simulink model "IEEE_39bus_load_increase_vol1"  (R2024b)
settings: Solver=ode23tb  StartTime=0.0  StopTime=500  MaxStep=1/60  RelTol=1e-2  AbsTol=1e-1  EnableMultiTasking=on
PreLoadFcn:
  | NE39bus_data;
  | PSSMODEL=1;
  | LPSS=0;
  | WAPSS=0;
  | WAPSS2=0;
values from neighbouring files (symbols this model uses):
  deg = [19.62;0;2.466;4.423;3.398;5.698;8.494;2.181;7.784;-3.646]*pi/180    [main_39.m]
  ki_sapc = 0.02*2.5/4    (= 0.0125)    [main_39.m]
  kp = 5*ones(10,1)    [main_39.m]
  kp_sapc = 0.15*1.25    (= 0.1875)    [main_39.m]
  line = [     1	2	0.0035	0.0411	0.6987	0	100	345 ... (first row only)    [main_39.m]
  P_base = mac_con(:,3).*[0.5609;0.6011;0.6995;0.6432;0.5143;0.6634;0.5676;0.5897;0.8444;0.3464]    [main_39.m]
  P_cmd = [1.140 	1.060 	1.100 	1.120 	0	1.060 	1.115 	1.160 	1.175 	1.000 ]    [main_39.m]
  Pmax = [1.20; 1.10; 1.15; 1.15;1.10;1.10;1.15;1.20;1.20;1.00]    [main_39.m]
  Pmin = 2-Pmax    [main_39.m]
  s = 10    [main_39.m]
  ts_pi = 5    [main_39.m]
  Udc = 2*Bus(mac_con(:,2),2)*1e3    [main_39.m]
  V_m = [1.03;0.982;0.9831;0.9972;1.0123;1.0493;1.0635;1.0278;1.0265;1.048]*sqrt(2/3)    [main_39.m]
undefined symbols (not defined in the file or in its folder): D1, Delta
libraries: spsThreePhaseVIMeasurementLib x40, spsThreePhasePISectionLineLib x34, spsThreePhaseParallelRLCLoadLib x21, spsThreePhaseTransformerTwoWindingsLib x13, spsMeanLib x12, slpidlib x12, spsLoadFlowBusLib x10, spsPLL3phLib x10, spsPowerPositiveSequenceLib x10, spsDCVoltageSourceLib x10, simulink x10, spsUniversalBridgeLib x10
(part 2 of 4)

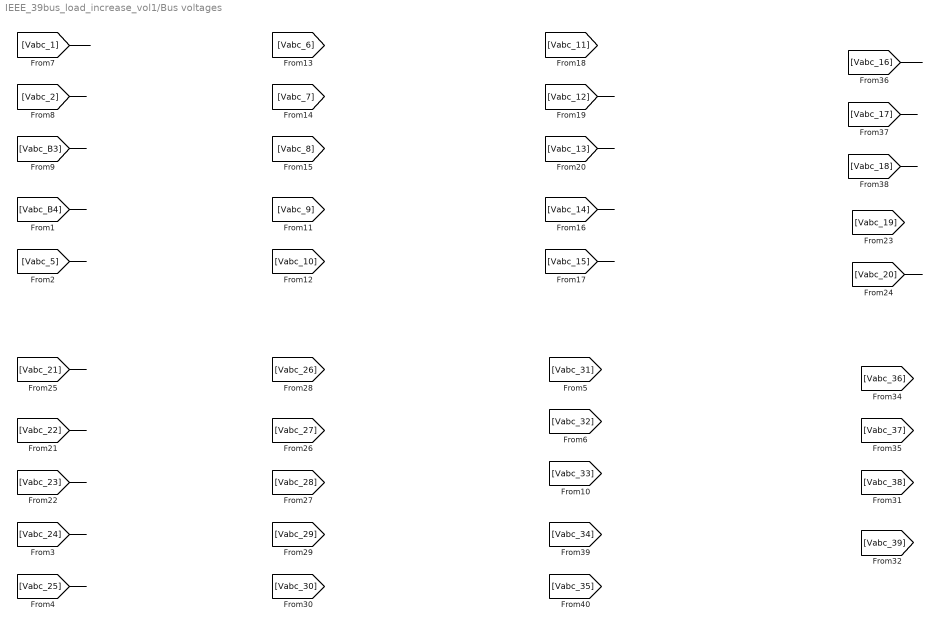
== system IEEE_39bus_load_increase_vol1/Bus voltages ==
  wires:
  [Vabc_1] -> ?
  [Vabc_2] -> ?
  [Vabc_B3] -> ?
  [Vabc_B4] -> ?
  [Vabc_5] -> ?
  [Vabc_24] -> ?
  [Vabc_25] -> ?
  [Vabc_12] -> ?
  [Vabc_13] -> ?
  [Vabc_14] -> ?
  [Vabc_15] -> ?
  [Vabc_20] -> ?
  [Vabc_21] -> ?
  [Vabc_22] -> ?
  [Vabc_23] -> ?
  [Vabc_16] -> ?
  [Vabc_17] -> ?
  [Vabc_18] -> ?

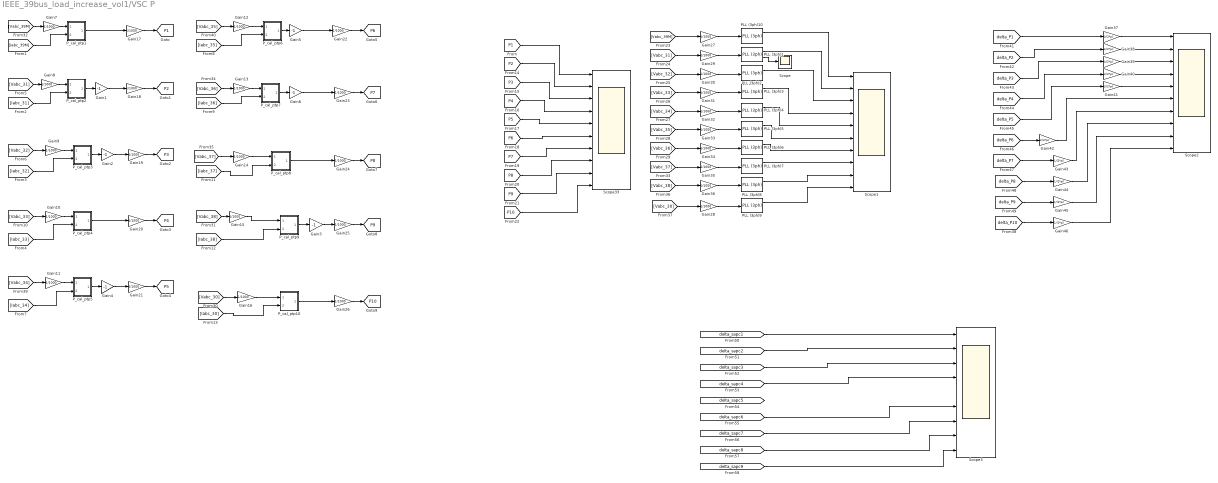
== system IEEE_39bus_load_increase_vol1/VSC P ==
  Gain{1..6} (6 alike) : Gain  Gain=-1
  Gain{7..36} (30 alike) : Gain  Gain=1/1000
  Gain{37..46} (10 alike) : Gain  Gain=1/(2*pi)
  PLL (3ph)1 : spsPLL3phLib/PLL (3ph)  Fmin=45  Par_Init=[deg(2)+30, 60]  ParK=[180, 3200, 1]/5  TcD=1e-4  MaxRateChangeFreq=200  FilterCutOffFreq=25  Ts=0  AGC=on
  PLL (3ph)10 : spsPLL3phLib/PLL (3ph)  Fmin=45  Par_Init=[deg(1)*180/pi+30, 60]  ParK=[180, 3200, 1]/5  TcD=1e-4  MaxRateChangeFreq=200  FilterCutOffFreq=25  Ts=0  AGC=on
  PLL (3ph)2 : spsPLL3phLib/PLL (3ph)  Fmin=45  Par_Init=[deg(3)*180/pi+30, 60]  ParK=[180, 3200, 1]/5  TcD=1e-4  MaxRateChangeFreq=200  FilterCutOffFreq=25  Ts=0  AGC=on
  PLL (3ph)3 : spsPLL3phLib/PLL (3ph)  Fmin=45  Par_Init=[deg(4)*180/pi+30, 60]  ParK=[180, 3200, 1]/5  TcD=1e-4  MaxRateChangeFreq=200  FilterCutOffFreq=25  Ts=0  AGC=on
  PLL (3ph)4 : spsPLL3phLib/PLL (3ph)  Fmin=45  Par_Init=[deg(5)*180/pi+30, 60]  ParK=[180, 3200, 1]/5  TcD=1e-4  MaxRateChangeFreq=200  FilterCutOffFreq=25  Ts=0  AGC=on
  PLL (3ph)5 : spsPLL3phLib/PLL (3ph)  Fmin=45  Par_Init=[deg(6)*180/pi+30, 60]  ParK=[180, 3200, 1]/5  TcD=1e-4  MaxRateChangeFreq=200  FilterCutOffFreq=25  Ts=0  AGC=on
  PLL (3ph)6 : spsPLL3phLib/PLL (3ph)  Fmin=45  Par_Init=[deg(7)*180/pi+30, 60]  ParK=[180, 3200, 1]/5  TcD=1e-4  MaxRateChangeFreq=200  FilterCutOffFreq=25  Ts=0  AGC=on
  PLL (3ph)7 : spsPLL3phLib/PLL (3ph)  Fmin=45  Par_Init=[deg(8)*180/pi+30, 60]  ParK=[180, 3200, 1]/5  TcD=1e-4  MaxRateChangeFreq=200  FilterCutOffFreq=25  Ts=0  AGC=on
  PLL (3ph)8 : spsPLL3phLib/PLL (3ph)  Fmin=45  Par_Init=[deg(9)*180/pi+30, 60]  ParK=[180, 3200, 1]/5  TcD=1e-4  MaxRateChangeFreq=200  FilterCutOffFreq=25  Ts=0  AGC=on
  PLL (3ph)9 : spsPLL3phLib/PLL (3ph)  Fmin=45  Par_Init=[deg(10)*180/pi+30, 60]  ParK=[180, 3200, 1]/5  TcD=1e-4  MaxRateChangeFreq=200  FilterCutOffFreq=25  Ts=0  AGC=on
  P_cal_ptp1 : Subsystem
  P_cal_ptp10 : Subsystem
  P_cal_ptp2 : Subsystem
  P_cal_ptp3 : Subsystem
  P_cal_ptp4 : Subsystem
  P_cal_ptp5 : Subsystem
  P_cal_ptp6 : Subsystem
  P_cal_ptp7 : Subsystem
  P_cal_ptp8 : Subsystem
  P_cal_ptp9 : Subsystem
  Scope : Scope
  Scope1 : Scope  NumInputPorts=10
  Scope2 : Scope  NumInputPorts=10
  Scope3 : Scope  NumInputPorts=9
  Scope33 : Scope  NumInputPorts=10
  tag scope: P10=global, P1=global, P2=global, P3=global, P4=global, P5=global, P6=global, P7=global, P8=global, P9=global
  wires:
  [Vabc_39M] -> Gain7/1
  [Iabc_39M] -> P_cal_ptp1/2(In1)
  [Vabc_31] -> Gain8/1
  [Iabc_31] -> P_cal_ptp2/2(In1)
  P_cal_ptp1/1(Out1) -> Gain17/1
  P_cal_ptp2/1(Out1) -> Gain1/1
  Gain1/1 -> Gain18/1
  [Vabc_32] -> Gain9/1
  P_cal_ptp3/1(Out1) -> Gain2/1
  [Iabc_32] -> P_cal_ptp3/2(In1)
  Gain2/1 -> Gain19/1
  [Vabc_33] -> Gain10/1
  [Iabc_33] -> P_cal_ptp4/2(In1)
  P_cal_ptp4/1(Out1) -> Gain20/1
  [Vabc_34] -> Gain11/1
  P_cal_ptp5/1(Out1) -> Gain4/1
  [Iabc_34] -> P_cal_ptp5/2(In1)
  Gain4/1 -> Gain21/1
  [Vabc_35] -> Gain12/1
  P_cal_ptp6/1(Out1) -> Gain5/1
  [Iabc_35] -> P_cal_ptp6/2(In1)
  Gain5/1 -> Gain22/1
  [Vabc_36] -> Gain13/1
  P_cal_ptp7/1(Out1) -> Gain6/1
  [Iabc_36] -> P_cal_ptp7/2(In1)
  Gain6/1 -> Gain23/1
  [Iabc_37] -> P_cal_ptp8/2(In1)
  [Vabc_37] -> Gain14/1
  P_cal_ptp8/1(Out1) -> Gain24/1
  [Vabc_38] -> Gain15/1
  [Iabc_38] -> P_cal_ptp9/2(In1)
  P_cal_ptp10/1(Out1) -> Gain26/1
  [Vabc_30] -> Gain16/1
  [Iabc_30] -> P_cal_ptp10/2(In1)
  [P1] -> Scope33/1
  [P2] -> Scope33/2
  [P3] -> Scope33/3
  [P4] -> Scope33/4
  [P5] -> Scope33/5
  [P6] -> Scope33/6
  [P7] -> Scope33/7
  [P8] -> Scope33/8
  [P9] -> Scope33/9
  [P10] -> Scope33/10
  P_cal_ptp9/1(Out1) -> Gain3/1
  Gain3/1 -> Gain25/1
  PLL (3ph)10/1 -> Scope1/1
  [Vabc_39M] -> Gain27/1
  [Vabc_31] -> Gain29/1
  PLL (3ph)1/1 -> Scope1/2
  [Vabc_32] -> Gain30/1
  PLL (3ph)2/1 -> Scope1/3
  [Vabc_33] -> Gain31/1
  PLL (3ph)3/1 -> Scope1/4
  [Vabc_34] -> Gain32/1
  PLL (3ph)4/1 -> Scope1/5
  [Vabc_35] -> Gain33/1
  PLL (3ph)5/1 -> Scope1/6
  [Vabc_36] -> Gain34/1
  PLL (3ph)6/1 -> Scope1/7
  [Vabc_37] -> Gain35/1
  PLL (3ph)7/1 -> Scope1/8
  [Vabc_38] -> Gain36/1
  PLL (3ph)8/1 -> Scope1/9
  [Vabc_30] -> Gain28/1
  PLL (3ph)9/1 -> Scope1/10
  Gain7/1 -> P_cal_ptp1/1(In2)
  Gain8/1 -> P_cal_ptp2/1(In2)
  Gain9/1 -> P_cal_ptp3/1(In2)
  Gain10/1 -> P_cal_ptp4/1(In2)
  Gain11/1 -> P_cal_ptp5/1(In2)
  Gain12/1 -> P_cal_ptp6/1(In2)
  Gain13/1 -> P_cal_ptp7/1(In2)
  Gain14/1 -> P_cal_ptp8/1(In2)
  Gain15/1 -> P_cal_ptp9/1(In2)
  Gain16/1 -> P_cal_ptp10/1(In2)
  Gain17/1 -> [P1]
  Gain18/1 -> [P2]
  Gain19/1 -> [P3]
  Gain20/1 -> [P4]
  Gain21/1 -> [P5]
  Gain22/1 -> [P6]
  Gain23/1 -> [P7]
  Gain24/1 -> [P8]
  Gain25/1 -> [P9]
  Gain26/1 -> [P10]
  Gain27/1 -> PLL (3ph)10/1
  Gain28/1 -> PLL (3ph)9/1
  Gain29/1 -> PLL (3ph)1/1
  Gain30/1 -> PLL (3ph)2/1
  Gain31/1 -> PLL (3ph)3/1
  Gain32/1 -> PLL (3ph)4/1
  Gain33/1 -> PLL (3ph)5/1
  Gain34/1 -> PLL (3ph)6/1
  Gain35/1 -> PLL (3ph)7/1
  Gain36/1 -> PLL (3ph)8/1
  PLL (3ph)1/2 -> Scope/1
  [delta_P1] -> Gain37/1
  [delta_P2] -> Gain38/1
  [delta_P3] -> Gain39/1
  [delta_P4] -> Gain40/1
  [delta_P5] -> Gain41/1
  [delta_P6] -> Gain42/1
  [delta_P7] -> Gain43/1
  [delta_P8] -> Gain44/1
  [delta_P9] -> Gain45/1
  [delta_P10] -> Gain46/1
  Gain37/1 -> Scope2/1
  Gain38/1 -> Scope2/2
  Gain39/1 -> Scope2/3
  Gain40/1 -> Scope2/4
  Gain41/1 -> Scope2/5
  Gain42/1 -> Scope2/6
  Gain43/1 -> Scope2/7
  Gain44/1 -> Scope2/8
  Gain45/1 -> Scope2/9
  Gain46/1 -> Scope2/10
  [delta_sapc8] -> Scope3/8
  [delta_sapc7] -> Scope3/7
  [delta_sapc6] -> Scope3/6
  [delta_sapc4] -> Scope3/4
  [delta_sapc3] -> Scope3/3
  [delta_sapc2] -> Scope3/2
  [delta_sapc1] -> Scope3/1
  [delta_sapc9] -> Scope3/9

== system IEEE_39bus_load_increase_vol1/VSC1 ==
  Add1 : Sum
  Constant : Constant  Value=P_cmd(1)
  DC Voltage Source2 : spsDCVoltageSourceLib/DC Voltage Source  Amplitude=Udc(1)  Measurements=None
  Discrete Derivative : simulink/Discrete/Discrete Derivative  gainval=1.0  ICPrevScaledInput=0.0  OutMin=[]  OutMax=[]  OutDataType=fixdt(1, 16)  OutScaling=2^-10  DoSatur=off
  Discrete Derivative1 : simulink/Discrete/Discrete Derivative  gainval=1.0  ICPrevScaledInput=0.0  OutMin=[]  OutMax=[]  OutDataType=fixdt(1, 16)  OutScaling=2^-10  DoSatur=off
  Gain4 : Gain  Gain=1/P_base(1)
  Memory2 : Memory
  Rate Transition : RateTransition  OutPortSampleTime=Ts_fre
  Subsystem3 : Subsystem
  VSC1 : spsUniversalBridgeLib/Universal Bridge  Arms=3  SnubberResistance=1e5  SnubberCapacitance=inf  Device=Average-model based VSC  Ron=1e-3  Lon=0  ForwardVoltages="[  0  0  ]"  ForwardVoltage=0  GTOparameters=[ 10e-6 , 20e-6 ]  IGBTparameters=[ 1e-6 , 2e-6 ]  Measurements=None  Measurements_2=None  converterType=Rectifier
  sapc : Subsystem
  A : PMIOPort  Side=Left
  B : PMIOPort  Port=2  Side=Left
  C : PMIOPort  Port=3  Side=Left
  tag scope: delta_P1=global
  wires:
  Memory2/1 -> VSC1/1
  [P1] -> Subsystem3/1(P2)
  sapc/1(delta) -> Rate Transition/1, Subsystem3/2(delta)
  Subsystem3/1(Out1) -> Memory2/1
  Constant/1 -> sapc/1(In1)
  Gain4/1 -> sapc/2(In2)
  [P1] -> Gain4/1
  Add1/1 -> [delta_P1]
  Subsystem3/2(Out2) -> Add1/1
  Discrete Derivative/1 -> Add1/2
  Rate Transition/1 -> Discrete Derivative/1
  connections:
  VSC1/LConn2 -- B/RConn1
  VSC1/RConn1 -- DC Voltage Source2/RConn1
  VSC1/RConn2 -- DC Voltage Source2/LConn1
  VSC1/LConn1 -- A/RConn1
  VSC1/LConn3 -- C/RConn1

== system IEEE_39bus_load_increase_vol1/VSC2 ==
  Add1 : Sum
  Constant : Constant  Value=P_cmd(2)
  DC Voltage Source1 : spsDCVoltageSourceLib/DC Voltage Source  Amplitude=Udc(2)  Measurements=None
  Discrete Derivative : simulink/Discrete/Discrete Derivative  gainval=1.0  ICPrevScaledInput=0.0  OutMin=[]  OutMax=[]  OutDataType=fixdt(1, 16)  OutScaling=2^-10  DoSatur=off
  Gain4 : Gain  Gain=1/P_base(2)
  Memory1 : Memory
  Rate Transition : RateTransition  OutPortSampleTime=Ts_fre
  Subsystem1 : Subsystem
  VSC2 : spsUniversalBridgeLib/Universal Bridge  Arms=3  SnubberResistance=1e5  SnubberCapacitance=inf  Device=Average-model based VSC  Ron=1e-3  Lon=0  ForwardVoltages="[  0  0  ]"  ForwardVoltage=0  GTOparameters=[ 10e-6 , 20e-6 ]  IGBTparameters=[ 1e-6 , 2e-6 ]  Measurements=None  Measurements_2=None  converterType=Rectifier
  sapc : Subsystem
  A : PMIOPort  Side=Left
  B : PMIOPort  Port=2  Side=Left
  C : PMIOPort  Port=3  Side=Left
  tag scope: delta_P2=global
  wires:
  Subsystem1/1(Out1) -> Memory1/1
  sapc/1(delta) -> Rate Transition/1, Subsystem1/2(delta)
  [P2] -> Subsystem1/1(P2)
  Memory1/1 -> VSC2/1
  [P2] -> Gain4/1
  Gain4/1 -> sapc/2(In2)
  Constant/1 -> sapc/1(In1)
  Discrete Derivative/1 -> Add1/2
  Add1/1 -> [delta_P2]
  Subsystem1/2(Out2) -> Add1/1
  Rate Transition/1 -> Discrete Derivative/1
  connections:
  VSC2/LConn2 -- B/RConn1
  VSC2/RConn2 -- DC Voltage Source1/LConn1
  VSC2/RConn1 -- DC Voltage Source1/RConn1
  VSC2/LConn3 -- C/RConn1
  VSC2/LConn1 -- A/RConn1

== system IEEE_39bus_load_increase_vol1/VSC3 ==
  Add1 : Sum
  Constant : Constant  Value=P_cmd(3)
  DC Voltage Source3 : spsDCVoltageSourceLib/DC Voltage Source  Amplitude=Udc(3)  Measurements=None
  Discrete Derivative : simulink/Discrete/Discrete Derivative  gainval=1.0  ICPrevScaledInput=0.0  OutMin=[]  OutMax=[]  OutDataType=fixdt(1, 16)  OutScaling=2^-10  DoSatur=off
  Gain4 : Gain  Gain=1/P_base(3)
  Memory3 : Memory
  Rate Transition : RateTransition  OutPortSampleTime=Ts_fre
  Subsystem2 : Subsystem
  VSC3 : spsUniversalBridgeLib/Universal Bridge  Arms=3  SnubberResistance=1e5  SnubberCapacitance=inf  Device=Average-model based VSC  Ron=1e-3  Lon=0  ForwardVoltages="[  0  0  ]"  ForwardVoltage=0  GTOparameters=[ 10e-6 , 20e-6 ]  IGBTparameters=[ 1e-6 , 2e-6 ]  Measurements=None  Measurements_2=None  converterType=Rectifier
  sapc : Subsystem
  A : PMIOPort  Side=Left
  B : PMIOPort  Port=2  Side=Left
  C : PMIOPort  Port=3  Side=Left
  tag scope: delta_P3=global
  wires:
  Subsystem2/1(Out1) -> Memory3/1
  [P3] -> Subsystem2/1(P2)
  sapc/1(delta) -> Rate Transition/1, Subsystem2/2(delta)
  Memory3/1 -> VSC3/1
  Constant/1 -> sapc/1(In1)
  Gain4/1 -> sapc/2(In2)
  [P3] -> Gain4/1
  Discrete Derivative/1 -> Add1/2
  Subsystem2/2(Out2) -> Add1/1
  Add1/1 -> [delta_P3]
  Rate Transition/1 -> Discrete Derivative/1
  connections:
  VSC3/RConn2 -- DC Voltage Source3/LConn1
  VSC3/RConn1 -- DC Voltage Source3/RConn1
  VSC3/LConn1 -- A/RConn1
  VSC3/LConn2 -- B/RConn1
  VSC3/LConn3 -- C/RConn1

== system IEEE_39bus_load_increase_vol1/vsc10 ==
  DC Voltage Source4 : spsDCVoltageSourceLib/DC Voltage Source  Amplitude=Udc(10)  Measurements=None
  Memory4 : Memory
  Subsystem4 : Subsystem
  VSC8 : spsUniversalBridgeLib/Universal Bridge  Arms=3  SnubberResistance=1e5  SnubberCapacitance=inf  Device=Average-model based VSC  Ron=1e-3  Lon=0  ForwardVoltages="[  0  0  ]"  ForwardVoltage=0  GTOparameters=[ 10e-6 , 20e-6 ]  IGBTparameters=[ 1e-6 , 2e-6 ]  Measurements=None  Measurements_2=None  converterType=Rectifier
  Vref4 : Constant  Value=0
  A : PMIOPort  Side=Left
  B : PMIOPort  Port=2  Side=Left
  C : PMIOPort  Port=3  Side=Left
  tag scope: delta_P10=global
  wires:
  Subsystem4/1(Out1) -> Memory4/1
  Vref4/1 -> Subsystem4/2(delta)
  [P10] -> Subsystem4/1(P2)
  Memory4/1 -> VSC8/1
  Subsystem4/2(Out2) -> [delta_P10]
  connections:
  VSC8/LConn1 -- A/RConn1
  VSC8/RConn2 -- DC Voltage Source4/LConn1
  VSC8/RConn1 -- DC Voltage Source4/RConn1
  VSC8/LConn2 -- B/RConn1
  VSC8/LConn3 -- C/RConn1

== system IEEE_39bus_load_increase_vol1/vsc4 ==
  Add1 : Sum
  Constant : Constant  Value=P_cmd(4)
  DC Voltage Source4 : spsDCVoltageSourceLib/DC Voltage Source  Amplitude=Udc(4)  Measurements=None
  Discrete Derivative : simulink/Discrete/Discrete Derivative  gainval=1.0  ICPrevScaledInput=0.0  OutMin=[]  OutMax=[]  OutDataType=fixdt(1, 16)  OutScaling=2^-10  DoSatur=off
  Gain4 : Gain  Gain=1/P_base(4)
  Memory4 : Memory
  Rate Transition : RateTransition  OutPortSampleTime=Ts_fre
  Subsystem4 : Subsystem
  VSC4 : spsUniversalBridgeLib/Universal Bridge  Arms=3  SnubberResistance=1e5  SnubberCapacitance=inf  Device=Average-model based VSC  Ron=1e-3  Lon=0  ForwardVoltages="[  0  0  ]"  ForwardVoltage=0  GTOparameters=[ 10e-6 , 20e-6 ]  IGBTparameters=[ 1e-6 , 2e-6 ]  Measurements=None  Measurements_2=None  converterType=Rectifier
  sapc : Subsystem
  A : PMIOPort  Side=Left
  B : PMIOPort  Port=2  Side=Left
  C : PMIOPort  Port=3  Side=Left
  tag scope: delta_P4=global
  wires:
  Subsystem4/1(Out1) -> Memory4/1
  [P4] -> Subsystem4/1(P2)
  Memory4/1 -> VSC4/1
  Constant/1 -> sapc/1(In1)
  Gain4/1 -> sapc/2(In2)
  [P4] -> Gain4/1
  sapc/1(delta) -> Rate Transition/1, Subsystem4/2(delta)
  Subsystem4/2(Out2) -> Add1/1
  Add1/1 -> [delta_P4]
  Rate Transition/1 -> Discrete Derivative/1
  Discrete Derivative/1 -> Add1/2
  connections:
  VSC4/LConn1 -- A/RConn1
  VSC4/RConn2 -- DC Voltage Source4/LConn1
  VSC4/RConn1 -- DC Voltage Source4/RConn1
  VSC4/LConn2 -- B/RConn1
  VSC4/LConn3 -- C/RConn1

== system IEEE_39bus_load_increase_vol1/vsc5 ==
  Add1 : Sum
  Constant : Constant  Value=1.05
  Constant1 : Constant  Value=0
  DC Voltage Source4 : spsDCVoltageSourceLib/DC Voltage Source  Amplitude=Udc(5)  Measurements=None
  Discrete Derivative : simulink/Discrete/Discrete Derivative  gainval=1.0  ICPrevScaledInput=0.0  OutMin=[]  OutMax=[]  OutDataType=fixdt(1, 16)  OutScaling=2^-10  DoSatur=off
  Gain4 : Gain  Gain=1/P_base(5)
  Memory4 : Memory
  Rate Transition : RateTransition  OutPortSampleTime=Ts_fre
  Subsystem4 : Subsystem
  VSC5 : spsUniversalBridgeLib/Universal Bridge  Arms=3  SnubberResistance=1e5  SnubberCapacitance=inf  Device=Average-model based VSC  Ron=1e-3  Lon=0  ForwardVoltages="[  0  0  ]"  ForwardVoltage=0  GTOparameters=[ 10e-6 , 20e-6 ]  IGBTparameters=[ 1e-6 , 2e-6 ]  Measurements=None  Measurements_2=None  converterType=Rectifier
  sapc : Subsystem
  A : PMIOPort  Side=Left
  B : PMIOPort  Port=2  Side=Left
  C : PMIOPort  Port=3  Side=Left
  tag scope: delta_P5=global
  wires:
  Subsystem4/1(Out1) -> Memory4/1
  [P5] -> Subsystem4/1(P2)
  Memory4/1 -> VSC5/1
  Gain4/1 -> sapc/2(In2)
  Constant/1 -> sapc/1(In1)
  [P5] -> Gain4/1
  Discrete Derivative/1 -> Add1/2
  Subsystem4/2(Out2) -> [delta_P5], Add1/1
  sapc/1(delta) -> Rate Transition/1
  Rate Transition/1 -> Discrete Derivative/1
  Constant1/1 -> Subsystem4/2(delta)
  connections:
  VSC5/LConn1 -- A/RConn1
  VSC5/RConn2 -- DC Voltage Source4/LConn1
  VSC5/RConn1 -- DC Voltage Source4/RConn1
  VSC5/LConn2 -- B/RConn1
  VSC5/LConn3 -- C/RConn1

== system IEEE_39bus_load_increase_vol1/vsc6 ==
  Add1 : Sum
  Constant : Constant  Value=P_cmd(6)
  DC Voltage Source4 : spsDCVoltageSourceLib/DC Voltage Source  Amplitude=Udc(6)  Measurements=None
  Discrete Derivative : simulink/Discrete/Discrete Derivative  gainval=1.0  ICPrevScaledInput=0.0  OutMin=[]  OutMax=[]  OutDataType=fixdt(1, 16)  OutScaling=2^-10  DoSatur=off
  Gain4 : Gain  Gain=1/P_base(6)
  Memory4 : Memory
  Rate Transition : RateTransition  OutPortSampleTime=Ts_fre
  Subsystem4 : Subsystem
  VSC6 : spsUniversalBridgeLib/Universal Bridge  Arms=3  SnubberResistance=1e5  SnubberCapacitance=inf  Device=Average-model based VSC  Ron=1e-3  Lon=0  ForwardVoltages="[  0  0  ]"  ForwardVoltage=0  GTOparameters=[ 10e-6 , 20e-6 ]  IGBTparameters=[ 1e-6 , 2e-6 ]  Measurements=None  Measurements_2=None  converterType=Rectifier
  sapc : Subsystem
  sapc1 : Subsystem
  A : PMIOPort  Side=Left
  B : PMIOPort  Port=2  Side=Left
  C : PMIOPort  Port=3  Side=Left
  tag scope: delta_P6=global
  wires:
  Subsystem4/1(Out1) -> Memory4/1
  [P6] -> Subsystem4/1(P2)
  Memory4/1 -> VSC6/1
  Gain4/1 -> sapc1/2(In2), sapc/2(In2)
  Constant/1 -> sapc/1(In1), sapc1/1(In1)
  [P6] -> Gain4/1
  Discrete Derivative/1 -> Add1/2
  Add1/1 -> [delta_P6]
  Subsystem4/2(Out2) -> Add1/1
  Rate Transition/1 -> Discrete Derivative/1
  sapc1/1(delta) -> Rate Transition/1, Subsystem4/2(delta)
  connections:
  VSC6/LConn1 -- A/RConn1
  VSC6/RConn2 -- DC Voltage Source4/LConn1
  VSC6/RConn1 -- DC Voltage Source4/RConn1
  VSC6/LConn2 -- B/RConn1
  VSC6/LConn3 -- C/RConn1

== system IEEE_39bus_load_increase_vol1/vsc7 ==
  Add1 : Sum
  Constant : Constant  Value=P_cmd(7)
  DC Voltage Source4 : spsDCVoltageSourceLib/DC Voltage Source  Amplitude=Udc(7)  Measurements=None
  Discrete Derivative : simulink/Discrete/Discrete Derivative  gainval=1.0  ICPrevScaledInput=0.0  OutMin=[]  OutMax=[]  OutDataType=fixdt(1, 16)  OutScaling=2^-10  DoSatur=off
  Gain4 : Gain  Gain=1/P_base(7)
  Memory4 : Memory
  Rate Transition : RateTransition  OutPortSampleTime=Ts_fre
  Subsystem4 : Subsystem
  VSC7 : spsUniversalBridgeLib/Universal Bridge  Arms=3  SnubberResistance=1e5  SnubberCapacitance=inf  Device=Average-model based VSC  Ron=1e-3  Lon=0  ForwardVoltages="[  0  0  ]"  ForwardVoltage=0  GTOparameters=[ 10e-6 , 20e-6 ]  IGBTparameters=[ 1e-6 , 2e-6 ]  Measurements=None  Measurements_2=None  converterType=Rectifier
  sapc : Subsystem
  sapc1 : Subsystem
  A : PMIOPort  Side=Left
  B : PMIOPort  Port=2  Side=Left
  C : PMIOPort  Port=3  Side=Left
  tag scope: delta_P7=global
  wires:
  Subsystem4/1(Out1) -> Memory4/1
  [P7] -> Subsystem4/1(P2)
  Memory4/1 -> VSC7/1
  Gain4/1 -> sapc1/2(In2), sapc/2(In2)
  Constant/1 -> sapc/1(In1), sapc1/1(In1)
  [P7] -> Gain4/1
  Rate Transition/1 -> Discrete Derivative/1
  Add1/1 -> [delta_P7]
  Subsystem4/2(Out2) -> Add1/1
  Discrete Derivative/1 -> Add1/2
  sapc1/1(delta) -> Rate Transition/1, Subsystem4/2(delta)
  connections:
  VSC7/LConn1 -- A/RConn1
  VSC7/RConn2 -- DC Voltage Source4/LConn1
  VSC7/RConn1 -- DC Voltage Source4/RConn1
  VSC7/LConn2 -- B/RConn1
  VSC7/LConn3 -- C/RConn1

== system IEEE_39bus_load_increase_vol1/vsc8 ==
  Add1 : Sum
  Constant : Constant  Value=P_cmd(8)
  DC Voltage Source4 : spsDCVoltageSourceLib/DC Voltage Source  Amplitude=Udc(8)  Measurements=None
  Discrete Derivative : simulink/Discrete/Discrete Derivative  gainval=1.0  ICPrevScaledInput=0.0  OutMin=[]  OutMax=[]  OutDataType=fixdt(1, 16)  OutScaling=2^-10  DoSatur=off
  Gain4 : Gain  Gain=1/P_base(8)
  Memory4 : Memory
  Rate Transition : RateTransition  OutPortSampleTime=Ts_fre
  Subsystem4 : Subsystem
  VSC8 : spsUniversalBridgeLib/Universal Bridge  Arms=3  SnubberResistance=1e5  SnubberCapacitance=inf  Device=Average-model based VSC  Ron=1e-3  Lon=0  ForwardVoltages="[  0  0  ]"  ForwardVoltage=0  GTOparameters=[ 10e-6 , 20e-6 ]  IGBTparameters=[ 1e-6 , 2e-6 ]  Measurements=None  Measurements_2=None  converterType=Rectifier
  sapc : Subsystem
  sapc1 : Subsystem
  A : PMIOPort  Side=Left
  B : PMIOPort  Port=2  Side=Left
  C : PMIOPort  Port=3  Side=Left
  tag scope: delta_P8=global
  wires:
  Subsystem4/1(Out1) -> Memory4/1
  [P8] -> Subsystem4/1(P2)
  Memory4/1 -> VSC8/1
  [P8] -> Gain4/1
  Constant/1 -> sapc1/1(In1), sapc/1(In1)
  Gain4/1 -> sapc1/2(In2), sapc/2(In2)
  Rate Transition/1 -> Discrete Derivative/1
  Add1/1 -> [delta_P8]
  Subsystem4/2(Out2) -> Add1/1
  Discrete Derivative/1 -> Add1/2
  sapc1/1(delta) -> Subsystem4/2(delta), Rate Transition/1
  connections:
  VSC8/LConn1 -- A/RConn1
  VSC8/RConn2 -- DC Voltage Source4/LConn1
  VSC8/RConn1 -- DC Voltage Source4/RConn1
  VSC8/LConn2 -- B/RConn1
  VSC8/LConn3 -- C/RConn1

== system IEEE_39bus_load_increase_vol1/vsc9 ==
  Add1 : Sum
  Constant : Constant  Value=P_cmd(9)
  Constant1 : Constant  Value=0
  DC Voltage Source4 : spsDCVoltageSourceLib/DC Voltage Source  Amplitude=Udc(9)  Measurements=None
  Discrete Derivative : simulink/Discrete/Discrete Derivative  gainval=1.0  ICPrevScaledInput=0.0  OutMin=[]  OutMax=[]  OutDataType=fixdt(1, 16)  OutScaling=2^-10  DoSatur=off
  Gain4 : Gain  Gain=1/P_base(9)
  Memory4 : Memory
  Rate Transition : RateTransition  OutPortSampleTime=Ts_fre
  Subsystem4 : Subsystem
  VSC5 : spsUniversalBridgeLib/Universal Bridge  Arms=3  SnubberResistance=1e5  SnubberCapacitance=inf  Device=Average-model based VSC  Ron=1e-3  Lon=0  ForwardVoltages="[  0  0  ]"  ForwardVoltage=0  GTOparameters=[ 10e-6 , 20e-6 ]  IGBTparameters=[ 1e-6 , 2e-6 ]  Measurements=None  Measurements_2=None  converterType=Rectifier
  sapc : Subsystem
  A : PMIOPort  Side=Left
  B : PMIOPort  Port=2  Side=Left
  C : PMIOPort  Port=3  Side=Left
  tag scope: delta_P9=global
  wires:
  Subsystem4/1(Out1) -> Memory4/1
  [P9] -> Subsystem4/1(P2)
  Memory4/1 -> VSC5/1
  [P9] -> Gain4/1
  Constant/1 -> sapc/1(In1)
  Gain4/1 -> sapc/2(In2)
  sapc/1(delta) -> Rate Transition/1, Subsystem4/2(delta)
  Rate Transition/1 -> Discrete Derivative/1
  Subsystem4/2(Out2) -> Add1/1
  Discrete Derivative/1 -> Add1/2
  Add1/1 -> [delta_P9]
  connections:
  VSC5/LConn1 -- A/RConn1
  VSC5/RConn2 -- DC Voltage Source4/LConn1
  VSC5/RConn1 -- DC Voltage Source4/RConn1
  VSC5/LConn2 -- B/RConn1
  VSC5/LConn3 -- C/RConn1

== system IEEE_39bus_load_increase_vol1/VSC P/P_cal_ptp1 ==
  In2 : Inport
  In1 : Inport  Port=2
  Add : Sum  Inputs=+++
  Demux1 : Demux  Outputs=3
  Demux2 : Demux  Outputs=3
  Gain1 : Gain  Gain=1/3
  Gain2 : Gain  Gain=1/3
  Gain3 : Gain  Gain=1/3
  Mean : spsMeanLib/Mean  Freq=60  Vinit=0  Ts=0
  Mux : Mux  Inputs=3
  Power (Positive-Sequence)1 : spsPowerPositiveSequenceLib/Power (Positive-Sequence)  Freq=60  Vinit=[0, 0]  Iinit=[0, 0]  Ts=1e-4
  Product : Product
  Product1 : Product
  Product2 : Product
  Sum : Sum  Inputs=|+-
  Sum1 : Sum  Inputs=|+-
  Sum2 : Sum  Inputs=|+-
  Out1 : Outport
  wires:
  Demux1/3 -> Sum1/1, Sum/2
  Mean/1 -> Out1/1
  In2/1 -> Demux2/1, Power (Positive-Sequence)1/1
  In1/1 -> Demux1/1
  Mux/1 -> Power (Positive-Sequence)1/2
  Demux1/1 -> Sum1/2, Sum2/1
  Demux1/2 -> Sum/1, Sum2/2
  Sum2/1 -> Gain2/1
  Sum/1 -> Gain1/1
  Sum1/1 -> Gain3/1
  Gain2/1 -> Product/2, Mux/1
  Gain1/1 -> Product1/2, Mux/2
  Gain3/1 -> Product2/2, Mux/3
  Product2/1 -> Add/3
  Product1/1 -> Add/2
  Product/1 -> Add/1
  Demux2/1 -> Product/1
  Demux2/2 -> Product1/1
  Demux2/3 -> Product2/1
  Power (Positive-Sequence)1/1 -> Mean/1

== system IEEE_39bus_load_increase_vol1/VSC P/P_cal_ptp10 ==
  In2 : Inport
  In1 : Inport  Port=2
  Add : Sum  Inputs=+++
  Demux1 : Demux  Outputs=3
  Demux2 : Demux  Outputs=3
  Gain1 : Gain  Gain=1/3
  Gain2 : Gain  Gain=1/3
  Gain3 : Gain  Gain=1/3
  Mean : spsMeanLib/Mean  Freq=60  Vinit=0  Ts=0
  Mux : Mux  Inputs=3
  Power (Positive-Sequence)1 : spsPowerPositiveSequenceLib/Power (Positive-Sequence)  Freq=60  Vinit=[0, 0]  Iinit=[0, 0]  Ts=1e-4
  Product : Product
  Product1 : Product
  Product2 : Product
  Sum : Sum  Inputs=|+-
  Sum1 : Sum  Inputs=|+-
  Sum2 : Sum  Inputs=|+-
  Out1 : Outport
  wires:
  Demux1/3 -> Sum1/1, Sum/2
  Mean/1 -> Out1/1
  In2/1 -> Demux2/1, Power (Positive-Sequence)1/1
  In1/1 -> Demux1/1
  Mux/1 -> Power (Positive-Sequence)1/2
  Demux1/1 -> Sum1/2, Sum2/1
  Demux1/2 -> Sum/1, Sum2/2
  Sum2/1 -> Gain2/1
  Sum/1 -> Gain1/1
  Sum1/1 -> Gain3/1
  Gain2/1 -> Product/2, Mux/1
  Gain1/1 -> Product1/2, Mux/2
  Gain3/1 -> Product2/2, Mux/3
  Product2/1 -> Add/3
  Product1/1 -> Add/2
  Product/1 -> Add/1
  Demux2/1 -> Product/1
  Demux2/2 -> Product1/1
  Demux2/3 -> Product2/1
  Power (Positive-Sequence)1/1 -> Mean/1

== system IEEE_39bus_load_increase_vol1/VSC P/P_cal_ptp2 ==
  In2 : Inport
  In1 : Inport  Port=2
  Add : Sum  Inputs=+++
  Demux1 : Demux  Outputs=3
  Demux2 : Demux  Outputs=3
  Gain1 : Gain  Gain=1/3
  Gain2 : Gain  Gain=1/3
  Gain3 : Gain  Gain=1/3
  Mean : spsMeanLib/Mean  Freq=60  Vinit=0  Ts=0
  Mux : Mux  Inputs=3
  Power (Positive-Sequence)1 : spsPowerPositiveSequenceLib/Power (Positive-Sequence)  Freq=60  Vinit=[0, 0]  Iinit=[0, 0]  Ts=1e-4
  Product : Product
  Product1 : Product
  Product2 : Product
  Sum : Sum  Inputs=|+-
  Sum1 : Sum  Inputs=|+-
  Sum2 : Sum  Inputs=|+-
  Out1 : Outport
  wires:
  Demux1/3 -> Sum1/1, Sum/2
  Mean/1 -> Out1/1
  In2/1 -> Demux2/1, Power (Positive-Sequence)1/1
  In1/1 -> Demux1/1
  Mux/1 -> Power (Positive-Sequence)1/2
  Demux1/1 -> Sum1/2, Sum2/1
  Demux1/2 -> Sum/1, Sum2/2
  Sum2/1 -> Gain2/1
  Sum/1 -> Gain1/1
  Sum1/1 -> Gain3/1
  Gain2/1 -> Product/2, Mux/1
  Gain1/1 -> Product1/2, Mux/2
  Gain3/1 -> Product2/2, Mux/3
  Product2/1 -> Add/3
  Product1/1 -> Add/2
  Product/1 -> Add/1
  Demux2/1 -> Product/1
  Demux2/2 -> Product1/1
  Demux2/3 -> Product2/1
  Power (Positive-Sequence)1/1 -> Mean/1

== system IEEE_39bus_load_increase_vol1/VSC P/P_cal_ptp3 ==
  In2 : Inport
  In1 : Inport  Port=2
  Add : Sum  Inputs=+++
  Demux1 : Demux  Outputs=3
  Demux2 : Demux  Outputs=3
  Gain1 : Gain  Gain=1/3
  Gain2 : Gain  Gain=1/3
  Gain3 : Gain  Gain=1/3
  Mean : spsMeanLib/Mean  Freq=60  Vinit=0  Ts=0
  Mux : Mux  Inputs=3
  Power (Positive-Sequence)1 : spsPowerPositiveSequenceLib/Power (Positive-Sequence)  Freq=60  Vinit=[0, 0]  Iinit=[0, 0]  Ts=1e-4
  Product : Product
  Product1 : Product
  Product2 : Product
  Sum : Sum  Inputs=|+-
  Sum1 : Sum  Inputs=|+-
  Sum2 : Sum  Inputs=|+-
  Out1 : Outport
  wires:
  Demux1/3 -> Sum1/1, Sum/2
  Mean/1 -> Out1/1
  In2/1 -> Demux2/1, Power (Positive-Sequence)1/1
  In1/1 -> Demux1/1
  Mux/1 -> Power (Positive-Sequence)1/2
  Demux1/1 -> Sum1/2, Sum2/1
  Demux1/2 -> Sum/1, Sum2/2
  Sum2/1 -> Gain2/1
  Sum/1 -> Gain1/1
  Sum1/1 -> Gain3/1
  Gain2/1 -> Product/2, Mux/1
  Gain1/1 -> Product1/2, Mux/2
  Gain3/1 -> Product2/2, Mux/3
  Product2/1 -> Add/3
  Product1/1 -> Add/2
  Product/1 -> Add/1
  Demux2/1 -> Product/1
  Demux2/2 -> Product1/1
  Demux2/3 -> Product2/1
  Power (Positive-Sequence)1/1 -> Mean/1

== system IEEE_39bus_load_increase_vol1/VSC P/P_cal_ptp4 ==
  In2 : Inport
  In1 : Inport  Port=2
  Add : Sum  Inputs=+++
  Demux1 : Demux  Outputs=3
  Demux2 : Demux  Outputs=3
  Gain1 : Gain  Gain=1/3
  Gain2 : Gain  Gain=1/3
  Gain3 : Gain  Gain=1/3
  Mean : spsMeanLib/Mean  Freq=60  Vinit=0  Ts=0
  Mux : Mux  Inputs=3
  Power (Positive-Sequence)1 : spsPowerPositiveSequenceLib/Power (Positive-Sequence)  Freq=60  Vinit=[0, 0]  Iinit=[0, 0]  Ts=1e-4
  Product : Product
  Product1 : Product
  Product2 : Product
  Sum : Sum  Inputs=|+-
  Sum1 : Sum  Inputs=|+-
  Sum2 : Sum  Inputs=|+-
  Out1 : Outport
  wires:
  Demux1/3 -> Sum1/1, Sum/2
  Mean/1 -> Out1/1
  In2/1 -> Demux2/1, Power (Positive-Sequence)1/1
  In1/1 -> Demux1/1
  Mux/1 -> Power (Positive-Sequence)1/2
  Demux1/1 -> Sum1/2, Sum2/1
  Demux1/2 -> Sum/1, Sum2/2
  Sum2/1 -> Gain2/1
  Sum/1 -> Gain1/1
  Sum1/1 -> Gain3/1
  Gain2/1 -> Product/2, Mux/1
  Gain1/1 -> Product1/2, Mux/2
  Gain3/1 -> Product2/2, Mux/3
  Product2/1 -> Add/3
  Product1/1 -> Add/2
  Product/1 -> Add/1
  Demux2/1 -> Product/1
  Demux2/2 -> Product1/1
  Demux2/3 -> Product2/1
  Power (Positive-Sequence)1/1 -> Mean/1

== system IEEE_39bus_load_increase_vol1/VSC P/P_cal_ptp5 ==
  In2 : Inport
  In1 : Inport  Port=2
  Add : Sum  Inputs=+++
  Demux1 : Demux  Outputs=3
  Demux2 : Demux  Outputs=3
  Gain1 : Gain  Gain=1/3
  Gain2 : Gain  Gain=1/3
  Gain3 : Gain  Gain=1/3
  Mean : spsMeanLib/Mean  Freq=60  Vinit=0  Ts=0
  Mux : Mux  Inputs=3
  Power (Positive-Sequence)1 : spsPowerPositiveSequenceLib/Power (Positive-Sequence)  Freq=60  Vinit=[0, 0]  Iinit=[0, 0]  Ts=1e-4
  Product : Product
  Product1 : Product
  Product2 : Product
  Sum : Sum  Inputs=|+-
  Sum1 : Sum  Inputs=|+-
  Sum2 : Sum  Inputs=|+-
  Out1 : Outport
  wires:
  Demux1/3 -> Sum1/1, Sum/2
  Mean/1 -> Out1/1
  In2/1 -> Demux2/1, Power (Positive-Sequence)1/1
  In1/1 -> Demux1/1
  Mux/1 -> Power (Positive-Sequence)1/2
  Demux1/1 -> Sum1/2, Sum2/1
  Demux1/2 -> Sum/1, Sum2/2
  Sum2/1 -> Gain2/1
  Sum/1 -> Gain1/1
  Sum1/1 -> Gain3/1
  Gain2/1 -> Product/2, Mux/1
  Gain1/1 -> Product1/2, Mux/2
  Gain3/1 -> Product2/2, Mux/3
  Product2/1 -> Add/3
  Product1/1 -> Add/2
  Product/1 -> Add/1
  Demux2/1 -> Product/1
  Demux2/2 -> Product1/1
  Demux2/3 -> Product2/1
  Power (Positive-Sequence)1/1 -> Mean/1

== system IEEE_39bus_load_increase_vol1/VSC P/P_cal_ptp6 ==
  In2 : Inport
  In1 : Inport  Port=2
  Add : Sum  Inputs=+++
  Demux1 : Demux  Outputs=3
  Demux2 : Demux  Outputs=3
  Gain1 : Gain  Gain=1/3
  Gain2 : Gain  Gain=1/3
  Gain3 : Gain  Gain=1/3
  Mean : spsMeanLib/Mean  Freq=60  Vinit=0  Ts=0
  Mux : Mux  Inputs=3
  Power (Positive-Sequence)1 : spsPowerPositiveSequenceLib/Power (Positive-Sequence)  Freq=60  Vinit=[0, 0]  Iinit=[0, 0]  Ts=1e-4
  Product : Product
  Product1 : Product
  Product2 : Product
  Sum : Sum  Inputs=|+-
  Sum1 : Sum  Inputs=|+-
  Sum2 : Sum  Inputs=|+-
  Out1 : Outport
  wires:
  Demux1/3 -> Sum1/1, Sum/2
  Mean/1 -> Out1/1
  In2/1 -> Demux2/1, Power (Positive-Sequence)1/1
  In1/1 -> Demux1/1
  Mux/1 -> Power (Positive-Sequence)1/2
  Demux1/1 -> Sum1/2, Sum2/1
  Demux1/2 -> Sum/1, Sum2/2
  Sum2/1 -> Gain2/1
  Sum/1 -> Gain1/1
  Sum1/1 -> Gain3/1
  Gain2/1 -> Product/2, Mux/1
  Gain1/1 -> Product1/2, Mux/2
  Gain3/1 -> Product2/2, Mux/3
  Product2/1 -> Add/3
  Product1/1 -> Add/2
  Product/1 -> Add/1
  Demux2/1 -> Product/1
  Demux2/2 -> Product1/1
  Demux2/3 -> Product2/1
  Power (Positive-Sequence)1/1 -> Mean/1

== system IEEE_39bus_load_increase_vol1/VSC P/P_cal_ptp7 ==
  In2 : Inport
  In1 : Inport  Port=2
  Add : Sum  Inputs=+++
  Demux1 : Demux  Outputs=3
  Demux2 : Demux  Outputs=3
  Gain1 : Gain  Gain=1/3
  Gain2 : Gain  Gain=1/3
  Gain3 : Gain  Gain=1/3
  Mean : spsMeanLib/Mean  Freq=60  Vinit=0  Ts=0
  Mux : Mux  Inputs=3
  Power (Positive-Sequence)1 : spsPowerPositiveSequenceLib/Power (Positive-Sequence)  Freq=60  Vinit=[0, 0]  Iinit=[0, 0]  Ts=1e-4
  Product : Product
  Product1 : Product
  Product2 : Product
  Sum : Sum  Inputs=|+-
  Sum1 : Sum  Inputs=|+-
  Sum2 : Sum  Inputs=|+-
  Out1 : Outport
  wires:
  Demux1/3 -> Sum1/1, Sum/2
  Mean/1 -> Out1/1
  In2/1 -> Demux2/1, Power (Positive-Sequence)1/1
  In1/1 -> Demux1/1
  Mux/1 -> Power (Positive-Sequence)1/2
  Demux1/1 -> Sum1/2, Sum2/1
  Demux1/2 -> Sum/1, Sum2/2
  Sum2/1 -> Gain2/1
  Sum/1 -> Gain1/1
  Sum1/1 -> Gain3/1
  Gain2/1 -> Product/2, Mux/1
  Gain1/1 -> Product1/2, Mux/2
  Gain3/1 -> Product2/2, Mux/3
  Product2/1 -> Add/3
  Product1/1 -> Add/2
  Product/1 -> Add/1
  Demux2/1 -> Product/1
  Demux2/2 -> Product1/1
  Demux2/3 -> Product2/1
  Power (Positive-Sequence)1/1 -> Mean/1

== system IEEE_39bus_load_increase_vol1/VSC P/P_cal_ptp8 ==
  In2 : Inport
  In1 : Inport  Port=2
  Add : Sum  Inputs=+++
  Demux1 : Demux  Outputs=3
  Demux2 : Demux  Outputs=3
  Gain1 : Gain  Gain=1/3
  Gain2 : Gain  Gain=1/3
  Gain3 : Gain  Gain=1/3
  Mean : spsMeanLib/Mean  Freq=60  Vinit=0  Ts=0
  Mux : Mux  Inputs=3
  Power (Positive-Sequence)1 : spsPowerPositiveSequenceLib/Power (Positive-Sequence)  Freq=60  Vinit=[0, 0]  Iinit=[0, 0]  Ts=1e-4
  Product : Product
  Product1 : Product
  Product2 : Product
  Sum : Sum  Inputs=|+-
  Sum1 : Sum  Inputs=|+-
  Sum2 : Sum  Inputs=|+-
  Out1 : Outport
  wires:
  Demux1/3 -> Sum1/1, Sum/2
  Mean/1 -> Out1/1
  In2/1 -> Demux2/1, Power (Positive-Sequence)1/1
  In1/1 -> Demux1/1
  Mux/1 -> Power (Positive-Sequence)1/2
  Demux1/1 -> Sum1/2, Sum2/1
  Demux1/2 -> Sum/1, Sum2/2
  Sum2/1 -> Gain2/1
  Sum/1 -> Gain1/1
  Sum1/1 -> Gain3/1
  Gain2/1 -> Product/2, Mux/1
  Gain1/1 -> Product1/2, Mux/2
  Gain3/1 -> Product2/2, Mux/3
  Product2/1 -> Add/3
  Product1/1 -> Add/2
  Product/1 -> Add/1
  Demux2/1 -> Product/1
  Demux2/2 -> Product1/1
  Demux2/3 -> Product2/1
  Power (Positive-Sequence)1/1 -> Mean/1

== system IEEE_39bus_load_increase_vol1/VSC P/P_cal_ptp9 ==
  In2 : Inport
  In1 : Inport  Port=2
  Add : Sum  Inputs=+++
  Demux1 : Demux  Outputs=3
  Demux2 : Demux  Outputs=3
  Gain1 : Gain  Gain=1/3
  Gain2 : Gain  Gain=1/3
  Gain3 : Gain  Gain=1/3
  Mean : spsMeanLib/Mean  Freq=60  Vinit=0  Ts=0
  Mux : Mux  Inputs=3
  Power (Positive-Sequence)1 : spsPowerPositiveSequenceLib/Power (Positive-Sequence)  Freq=60  Vinit=[0, 0]  Iinit=[0, 0]  Ts=1e-4
  Product : Product
  Product1 : Product
  Product2 : Product
  Sum : Sum  Inputs=|+-
  Sum1 : Sum  Inputs=|+-
  Sum2 : Sum  Inputs=|+-
  Out1 : Outport
  wires:
  Demux1/3 -> Sum1/1, Sum/2
  Mean/1 -> Out1/1
  In2/1 -> Demux2/1, Power (Positive-Sequence)1/1
  In1/1 -> Demux1/1
  Mux/1 -> Power (Positive-Sequence)1/2
  Demux1/1 -> Sum1/2, Sum2/1
  Demux1/2 -> Sum/1, Sum2/2
  Sum2/1 -> Gain2/1
  Sum/1 -> Gain1/1
  Sum1/1 -> Gain3/1
  Gain2/1 -> Product/2, Mux/1
  Gain1/1 -> Product1/2, Mux/2
  Gain3/1 -> Product2/2, Mux/3
  Product2/1 -> Add/3
  Product1/1 -> Add/2
  Product/1 -> Add/1
  Demux2/1 -> Product/1
  Demux2/2 -> Product1/1
  Demux2/3 -> Product2/1
  Power (Positive-Sequence)1/1 -> Mean/1

== system IEEE_39bus_load_increase_vol1/VSC1/Subsystem3 ==
  P2 : Inport
  delta : Inport  Port=2
  Add1 : Sum  Inputs=++++
  Clock1 : Clock
  Constant1 : Constant  Value="[0  -2/3*pi   2/3*pi]+deg(1)"
  Constant2 : Constant  Value=0
  Constant3 : Constant  Value=0
  Constant4 : Constant  Value=Pmax(1)
  Constant5 : Constant  Value=Pmin(1)
  Gain : Gain  Gain=kp(1)
  Gain1 : Gain  Gain=[1 1 1]
  Gain2 : Gain  Gain=120*pi*[1 1 1]
  Gain3 : Gain  Gain=V_m(1)
  Gain4 : Gain  Gain=1/P_base(1)
  Gain5 : Gain  Gain=[1 1 1]
  Gain6 : Gain  Gain=-1
  Integrator : Integrator
  Product : Product
  Product1 : Product
  Scope1 : Scope
  Scope2 : Scope
  Scope3 : Scope
  Step : Step  Time=5  SampleTime=0
  Step1 : Step  Time=5  SampleTime=0
  Sum : Sum  Inputs=|+-
  Sum1 : Sum  Inputs=|+-
  Sum2 : Sum  Inputs=|++
  Switch : Switch  Criteria=u2 > Threshold  Threshold=Pmax(1)  SaturateOnIntegerOverflow=off  InputSameDT=off
  Switch1 : Switch  Criteria=u2 > Threshold  Threshold=-Pmin(1)  SaturateOnIntegerOverflow=off  InputSameDT=off
  Trigonometric Function1 : Trigonometry
  Out1 : Outport
  Out2 : Outport  Port=2
  wires:
  Clock1/1 -> Gain2/1
  Constant1/1 -> Add1/2
  Gain2/1 -> Add1/1
  Add1/1 -> Trigonometric Function1/1
  Gain1/1 -> Product/1
  Step/1 -> Product/2
  Product/1 -> Add1/3
  Trigonometric Function1/1 -> Gain3/1
  Gain3/1 -> Out1/1
  P2/1 -> Gain4/1
  delta/1 -> Gain5/1
  Gain5/1 -> Add1/4
  Step1/1 -> Product1/2
  Constant4/1 -> Sum/1
  Sum/1 -> Switch/1
  Constant2/1 -> Switch/3
  Constant5/1 -> Sum1/1
  Sum1/1 -> Switch1/1
  Gain4/1 -> Gain6/1, Sum1/2, Sum/2, Switch/2
  Constant3/1 -> Switch1/3
  Gain6/1 -> Switch1/2
  Switch/1 -> Scope1/1, Sum2/1
  Switch1/1 -> Scope3/1, Sum2/2
  Sum2/1 -> Product1/1
  Product1/1 -> Gain/1
  Integrator/1 -> Gain1/1
  Gain/1 -> Scope2/1, Out2/1, Integrator/1

== system IEEE_39bus_load_increase_vol1/VSC1/sapc ==
  In1 : Inport
  In2 : Inport  Port=2
  Abs1 : Abs  SaturateOnIntegerOverflow=off
  Constant : Constant  Value=kp_sapc
  Constant1 : Constant  Value=ki_sapc
  Constant3 : Constant  Value=2
  Constant4 : Constant  Value=0.015
  Discrete PID Controller : slpidlib/PID Controller  Controller=PI  Form=Parallel  TimeDomain=Discrete-time  UseExternalTs=off  SampleTime=-1  IntegratorMethod=Forward Euler  FilterMethod=Forward Euler  ControllerParametersSource=external  P=kp_sapc*3  I=ki_sapc*2  UseKiTs=off  D=0  UseExternalDerivativeSource=off  N=100  UseFilter=on  TunerSelectOption=Transfer Function Based (PID Tuner App)  InitialConditionSource=internal  InitialConditionForIntegrator=0  InitialConditionForFilter=0  DifferentiatorICPrevScaledInput=0  ExternalReset=none  TrackingMode=off  Kt=1  LimitOutput=off  SatLimitsSource=internal  UpperSaturationLimit=inf  LowerSaturationLimit=-inf  LinearizeAsGain=off  AntiWindupMode=none  Kb=1  LimitIntegrator=off  UpperIntegratorSaturationLimit=inf  LowerIntegratorSaturationLimit=-inf  POutMin=[]  POutMax=[]  IOutMin=[]  IOutMax=[]  DOutMin=[]  DOutMax=[]  NOutMin=[]  NOutMax=[]  SumOutMin=[]  SumOutMax=[]  SaturationOutMin=[]  SaturationOutMax=[]  PParamMin=[]  PParamMax=[]  IParamMin=[]  IParamMax=[]  DParamMin=[]  DParamMax=[]  NParamMin=[]  NParamMax=[]  KbParamMin=[]  KbParamMax=[]  KtParamMin=[]  KtParamMax=[]  KbOutMin=[]  KbOutMax=[]  KtOutMin=[]  KtOutMax=[]  IntegratorOutMin=[]  IntegratorOutMax=[]  FilterOutMin=[]  FilterOutMax=[]  SumI1OutMin=[]  SumI1OutMax=[]  SumI2OutMin=[]  SumI2OutMax=[]  SumI3OutMin=[]  SumI3OutMax=[]  SumI4OutMin=[]  SumI4OutMax=[]  SumDOutMin=[]  SumDOutMax=[]  DifferentiatorOutMin=[]  DifferentiatorOutMax=[]  FilterDiffOutCoefMin=[]  FilterDiffOutCoefMax=[]  ReciprocalOutMin=[]  ReciprocalOutMax=[]  SumDenOutMin=[]  SumDenOutMax=[]  SumNumOutMin=[]  SumNumOutMax=[]  DivideOutMin=[]  DivideOutMax=[]  UdiffTsProdOutMin=[]  UdiffTsProdOutMax=[]  NTsProdOutMin=[]  NTsProdOutMax=[]  UintegralTsProdOutMin=[]  UintegralTsProdOutMax=[]  UngainTsProdOutMin=[]  UngainTsProdOutMax=[]  ClampingZeroOutDataTypeStr=Inherit: Inherit via back propagation  ClampingZeroOutMin=[]  ClampingZeroOutMax=[]  FilterDenConstantOutDataTypeStr=Inherit: Inherit via back propagation  FilterDenConstantOutMin=[]  FilterDenConstantOutMax=[]  PCopyOutDataTypeStr=Inherit: Inherit via back propagation  PCopyOutMin=[]  PCopyOutMax=[]  NCopyOutDataTypeStr=Inherit: Inherit via back propagation  NCopyOutMin=[]  NCopyOutMax=[]  IntegratorContinuousStateAttributes=''  IntegratorStateMustResolveToSignalObject=off  IntegratorRTWStateStorageClass=Auto  FilterContinuousStateAttributes=''  FilterStateMustResolveToSignalObject=off  FilterRTWStateStorageClass=Auto  ParallelPVariant=ExternalParameters  IdealPVariant=Disabled  IVariant=ExternalParameters  DVariant=Disabled  IntegratorVariant=Discrete  SatVariant=Disabled  AWVariant=Passthrough  PCopyVariant=Disabled  TRVariant=Disabled  FdbkBlocksVariant=Forward  IdealPFdbkVariant=Disabled  SatFdbkVariant=Disabled  DerivativeFilterVariant=Disabled  NVariant=Disabled  NCopyVariant=Disabled_SignalSpec  FilterICVariant=Disabled  IntegratorICVariant=InternalICs  ExternalResetVariant=Disabled  TRSumVariant=Passthrough  SumFdbkVariant=Disabled  SumVariant=Sum_PI  TsampFilterVariant=InternalTs  TsampNgainVariant=Passthrough  TsampIntegralVariant=Disabled_SignalSpec  ExternalSaturationOutDataTypeStr=Inherit: Same as second input  DerivativeSourceVariant=Disabled  PreIntVariant=InternalPreInt
      settings: LibrarySourceBlock=simulink/Discrete/Discrete PID Controller
  Gain1 : Gain  Gain=1/0.01/0.01
  Gain4 : Gain  Gain=P_base(1)/1e3
  Mean : spsMeanLib/Mean  Freq=5  Vinit=0  Ts=0
  Product{,1..3} (4 alike) : Product
  Saturation : Saturate  UpperLimit=3  LowerLimit=1
  Scope1 : Scope  NumInputPorts=2
  Scope2 : Scope  NumInputPorts=2
  Step : Step  Time=15  SampleTime=0
  Sum : Sum  Inputs=|+-
  Sum1 : Sum  Inputs=|+-
  Sum2 : Sum  Inputs=|+-
  Zero-Order Hold : ZeroOrderHold  SampleTime=ts_pi
  delta : Outport
  tag scope: delta_sapc1=global
  wires:
  Product/1 -> [delta_sapc1], Scope1/2, Discrete PID Controller/1
  Step/1 -> Product/2
  Sum/1 -> Gain4/1
  Discrete PID Controller/1 -> Scope1/1, Zero-Order Hold/1
  In1/1 -> Sum/1
  In2/1 -> Sum/2
  Zero-Order Hold/1 -> delta/1
  Constant/1 -> Product1/1
  Constant1/1 -> Product2/2
  Product2/1 -> Scope2/2, Discrete PID Controller/3
  Product1/1 -> Scope2/1, Discrete PID Controller/2
  Sum2/1 -> Saturation/1
  Saturation/1 -> Mean/1
  Gain4/1 -> Abs1/1, Product/1
  Abs1/1 -> Sum1/2
  Product3/1 -> Gain1/1
  Constant3/1 -> Sum2/1
  Constant4/1 -> Sum1/1
  Sum1/1 -> Product3/1, Product3/2
  Gain1/1 -> Sum2/2
  Mean/1 -> Product2/1, Product1/2

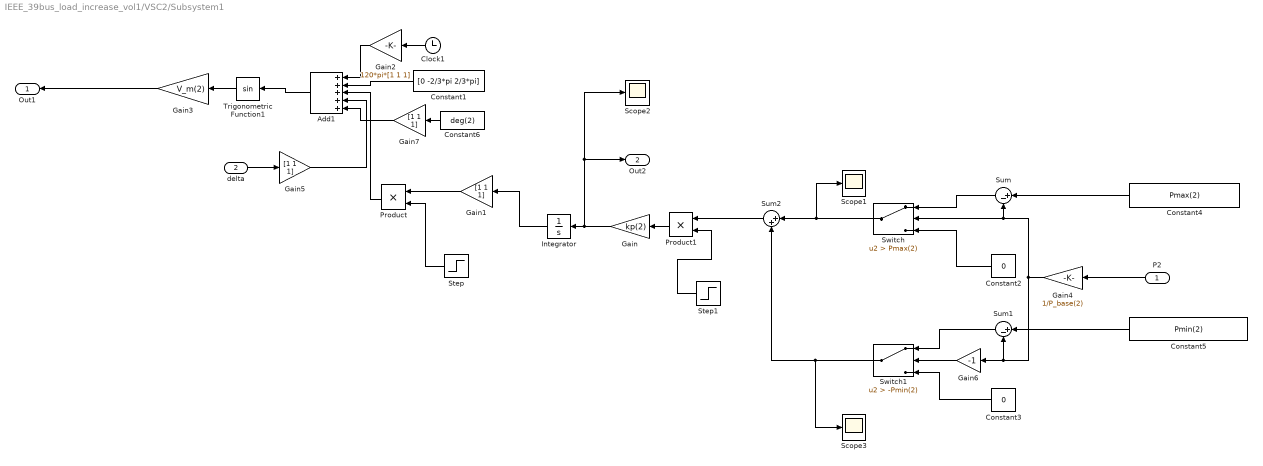
== system IEEE_39bus_load_increase_vol1/VSC2/Subsystem1 ==
  P2 : Inport
  delta : Inport  Port=2
  Add1 : Sum  Inputs=+++++
  Clock1 : Clock
  Constant1 : Constant  Value="[0  -2/3*pi   2/3*pi]"
  Constant2 : Constant  Value=0
  Constant3 : Constant  Value=0
  Constant4 : Constant  Value=Pmax(2)
  Constant5 : Constant  Value=Pmin(2)
  Constant6 : Constant  Value=deg(2)
  Gain : Gain  Gain=kp(2)
  Gain1 : Gain  Gain=[1 1 1]
  Gain2 : Gain  Gain=120*pi*[1 1 1]
  Gain3 : Gain  Gain=V_m(2)
  Gain4 : Gain  Gain=1/P_base(2)
  Gain5 : Gain  Gain=[1 1 1]
  Gain6 : Gain  Gain=-1
  Gain7 : Gain  Gain=[1 1 1]
  Integrator : Integrator
  Product : Product
  Product1 : Product
  Scope1 : Scope
  Scope2 : Scope
  Scope3 : Scope
  Step : Step  Time=5  SampleTime=0
  Step1 : Step  Time=5  SampleTime=0
  Sum : Sum  Inputs=|+-
  Sum1 : Sum  Inputs=|+-
  Sum2 : Sum  Inputs=|++
  Switch : Switch  Criteria=u2 > Threshold  Threshold=Pmax(2)  SaturateOnIntegerOverflow=off  InputSameDT=off
  Switch1 : Switch  Criteria=u2 > Threshold  Threshold=-Pmin(2)  SaturateOnIntegerOverflow=off  InputSameDT=off
  Trigonometric Function1 : Trigonometry
  Out1 : Outport
  Out2 : Outport  Port=2
  wires:
  Clock1/1 -> Gain2/1
  Constant1/1 -> Add1/2
  Gain2/1 -> Add1/1
  Add1/1 -> Trigonometric Function1/1
  Gain1/1 -> Product/1
  Step/1 -> Product/2
  Product/1 -> Add1/3
  Trigonometric Function1/1 -> Gain3/1
  Gain3/1 -> Out1/1
  P2/1 -> Gain4/1
  delta/1 -> Gain5/1
  Gain5/1 -> Add1/4
  Step1/1 -> Product1/2
  Constant4/1 -> Sum/1
  Sum/1 -> Switch/1
  Constant2/1 -> Switch/3
  Constant5/1 -> Sum1/1
  Sum1/1 -> Switch1/1
  Gain4/1 -> Gain6/1, Sum1/2, Sum/2, Switch/2
  Constant3/1 -> Switch1/3
  Gain6/1 -> Switch1/2
  Switch/1 -> Scope1/1, Sum2/1
  Switch1/1 -> Scope3/1, Sum2/2
  Sum2/1 -> Product1/1
  Constant6/1 -> Gain7/1
  Gain7/1 -> Add1/5
  Product1/1 -> Gain/1
  Gain/1 -> Out2/1, Scope2/1, Integrator/1
  Integrator/1 -> Gain1/1

== system IEEE_39bus_load_increase_vol1/VSC2/sapc ==
  In1 : Inport
  In2 : Inport  Port=2
  Abs1 : Abs  SaturateOnIntegerOverflow=off
  Constant : Constant  Value=kp_sapc
  Constant1 : Constant  Value=ki_sapc
  Constant2 : Constant  Value=1/0.015
  Constant3 : Constant  Value=2
  Constant4 : Constant  Value=0.01
  Delay2 : Delay  DelayLength=1  InitialCondition=0  SampleTime=1e-4
  Discrete PID Controller : slpidlib/PID Controller  Controller=PI  Form=Parallel  TimeDomain=Discrete-time  UseExternalTs=off  SampleTime=-1  IntegratorMethod=Forward Euler  FilterMethod=Forward Euler  ControllerParametersSource=external  P=kp_sapc*2  I=ki_sapc*2  UseKiTs=off  D=0  UseExternalDerivativeSource=off  N=100  UseFilter=on  TunerSelectOption=Transfer Function Based (PID Tuner App)  InitialConditionSource=internal  InitialConditionForIntegrator=0  InitialConditionForFilter=0  DifferentiatorICPrevScaledInput=0  ExternalReset=none  TrackingMode=off  Kt=1  LimitOutput=off  SatLimitsSource=internal  UpperSaturationLimit=inf  LowerSaturationLimit=-inf  LinearizeAsGain=off  AntiWindupMode=none  Kb=1  LimitIntegrator=off  UpperIntegratorSaturationLimit=inf  LowerIntegratorSaturationLimit=-inf  POutMin=[]  POutMax=[]  IOutMin=[]  IOutMax=[]  DOutMin=[]  DOutMax=[]  NOutMin=[]  NOutMax=[]  SumOutMin=[]  SumOutMax=[]  SaturationOutMin=[]  SaturationOutMax=[]  PParamMin=[]  PParamMax=[]  IParamMin=[]  IParamMax=[]  DParamMin=[]  DParamMax=[]  NParamMin=[]  NParamMax=[]  KbParamMin=[]  KbParamMax=[]  KtParamMin=[]  KtParamMax=[]  KbOutMin=[]  KbOutMax=[]  KtOutMin=[]  KtOutMax=[]  IntegratorOutMin=[]  IntegratorOutMax=[]  FilterOutMin=[]  FilterOutMax=[]  SumI1OutMin=[]  SumI1OutMax=[]  SumI2OutMin=[]  SumI2OutMax=[]  SumI3OutMin=[]  SumI3OutMax=[]  SumI4OutMin=[]  SumI4OutMax=[]  SumDOutMin=[]  SumDOutMax=[]  DifferentiatorOutMin=[]  DifferentiatorOutMax=[]  FilterDiffOutCoefMin=[]  FilterDiffOutCoefMax=[]  ReciprocalOutMin=[]  ReciprocalOutMax=[]  SumDenOutMin=[]  SumDenOutMax=[]  SumNumOutMin=[]  SumNumOutMax=[]  DivideOutMin=[]  DivideOutMax=[]  UdiffTsProdOutMin=[]  UdiffTsProdOutMax=[]  NTsProdOutMin=[]  NTsProdOutMax=[]  UintegralTsProdOutMin=[]  UintegralTsProdOutMax=[]  UngainTsProdOutMin=[]  UngainTsProdOutMax=[]  ClampingZeroOutDataTypeStr=Inherit: Inherit via back propagation  ClampingZeroOutMin=[]  ClampingZeroOutMax=[]  FilterDenConstantOutDataTypeStr=Inherit: Inherit via back propagation  FilterDenConstantOutMin=[]  FilterDenConstantOutMax=[]  PCopyOutDataTypeStr=Inherit: Inherit via back propagation  PCopyOutMin=[]  PCopyOutMax=[]  NCopyOutDataTypeStr=Inherit: Inherit via back propagation  NCopyOutMin=[]  NCopyOutMax=[]  IntegratorContinuousStateAttributes=''  IntegratorStateMustResolveToSignalObject=off  IntegratorRTWStateStorageClass=Auto  FilterContinuousStateAttributes=''  FilterStateMustResolveToSignalObject=off  FilterRTWStateStorageClass=Auto  ParallelPVariant=ExternalParameters  IdealPVariant=Disabled  IVariant=ExternalParameters  DVariant=Disabled  IntegratorVariant=Discrete  SatVariant=Disabled  AWVariant=Passthrough  PCopyVariant=Disabled  TRVariant=Disabled  FdbkBlocksVariant=Forward  IdealPFdbkVariant=Disabled  SatFdbkVariant=Disabled  DerivativeFilterVariant=Disabled  NVariant=Disabled  NCopyVariant=Disabled_SignalSpec  FilterICVariant=Disabled  IntegratorICVariant=InternalICs  ExternalResetVariant=Disabled  TRSumVariant=Passthrough  SumFdbkVariant=Disabled  SumVariant=Sum_PI  TsampFilterVariant=InternalTs  TsampNgainVariant=Passthrough  TsampIntegralVariant=Disabled_SignalSpec  ExternalSaturationOutDataTypeStr=Inherit: Same as second input  DerivativeSourceVariant=Disabled  PreIntVariant=InternalPreInt
      settings: LibrarySourceBlock=simulink/Discrete/Discrete PID Controller
  Gain1 : Gain  Gain=1/0.01/0.005
  Gain2 : Gain  Gain=1/2
  Gain4 : Gain  Gain=P_base(2)/1e3
  Product{,1..5} (6 alike) : Product
  Saturation : Saturate  UpperLimit=1  LowerLimit=1
  Saturation1 : Saturate  UpperLimit=1  LowerLimit=0
  Scope1 : Scope  NumInputPorts=3
  Scope2 : Scope  NumInputPorts=2
  Step : Step  Time=15  SampleTime=0
  Sum : Sum  Inputs=|+-
  Sum1 : Sum  Inputs=|+-
  Sum2 : Sum  Inputs=|+-
  Sum3 : Sum  Inputs=|++
  Zero-Order Hold : ZeroOrderHold  SampleTime=ts_pi
  delta : Outport
  tag scope: delta_sapc2=global
  wires:
  Product/1 -> [delta_sapc2], Scope1/3, Discrete PID Controller/1
  Step/1 -> Product/2
  Sum/1 -> Gain4/1
  Discrete PID Controller/1 -> Scope1/1, Zero-Order Hold/1
  In1/1 -> Sum/1
  In2/1 -> Sum/2
  Zero-Order Hold/1 -> Scope1/2, delta/1
  Constant1/1 -> Product2/2
  Constant/1 -> Product1/1
  Product2/1 -> Scope2/2, Discrete PID Controller/3
  Product1/1 -> Scope2/1, Discrete PID Controller/2
  Saturation/1 -> Product2/1, Product1/2
  Constant4/1 -> Sum1/1
  Abs1/1 -> Product5/2, Sum1/2
  Constant3/1 -> Sum2/1
  Product3/1 -> Gain1/1
  Gain1/1 -> Sum2/2
  Gain4/1 -> Abs1/1, Product/1
  Sum2/1 -> Product4/2
  Product5/1 -> Saturation1/1
  Sum1/1 -> Product3/1, Product3/2
  Constant2/1 -> Product5/1
  Saturation1/1 -> Product4/1
  Delay2/1 -> Sum3/1
  Product4/1 -> Sum3/2, Delay2/1
  Gain2/1 -> Saturation/1
  Sum3/1 -> Gain2/1

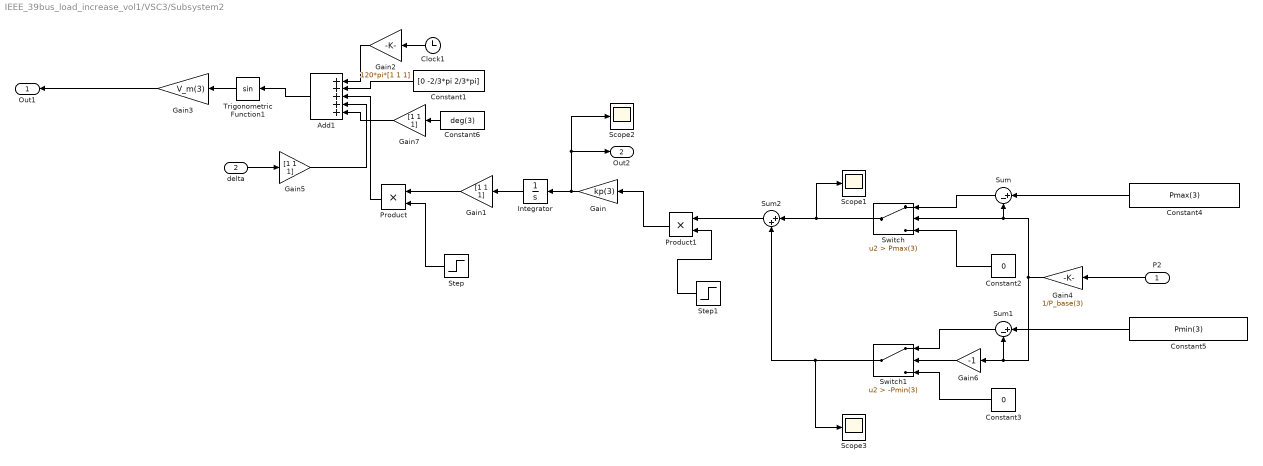
== system IEEE_39bus_load_increase_vol1/VSC3/Subsystem2 ==
  P2 : Inport
  delta : Inport  Port=2
  Add1 : Sum  Inputs=+++++
  Clock1 : Clock
  Constant1 : Constant  Value="[0  -2/3*pi   2/3*pi]"
  Constant2 : Constant  Value=0
  Constant3 : Constant  Value=0
  Constant4 : Constant  Value=Pmax(3)
  Constant5 : Constant  Value=Pmin(3)
  Constant6 : Constant  Value=deg(3)
  Gain : Gain  Gain=kp(3)
  Gain1 : Gain  Gain=[1 1 1]
  Gain2 : Gain  Gain=120*pi*[1 1 1]
  Gain3 : Gain  Gain=V_m(3)
  Gain4 : Gain  Gain=1/P_base(3)
  Gain5 : Gain  Gain=[1 1 1]
  Gain6 : Gain  Gain=-1
  Gain7 : Gain  Gain=[1 1 1]
  Integrator : Integrator
  Product : Product
  Product1 : Product
  Scope1 : Scope
  Scope2 : Scope
  Scope3 : Scope
  Step : Step  Time=5  SampleTime=0
  Step1 : Step  Time=5  SampleTime=0
  Sum : Sum  Inputs=|+-
  Sum1 : Sum  Inputs=|+-
  Sum2 : Sum  Inputs=|++
  Switch : Switch  Criteria=u2 > Threshold  Threshold=Pmax(3)  SaturateOnIntegerOverflow=off  InputSameDT=off
  Switch1 : Switch  Criteria=u2 > Threshold  Threshold=-Pmin(3)  SaturateOnIntegerOverflow=off  InputSameDT=off
  Trigonometric Function1 : Trigonometry
  Out1 : Outport
  Out2 : Outport  Port=2
  wires:
  Clock1/1 -> Gain2/1
  Constant1/1 -> Add1/2
  Gain2/1 -> Add1/1
  Add1/1 -> Trigonometric Function1/1
  Gain1/1 -> Product/1
  Step/1 -> Product/2
  Product/1 -> Add1/3
  Trigonometric Function1/1 -> Gain3/1
  Gain3/1 -> Out1/1
  P2/1 -> Gain4/1
  delta/1 -> Gain5/1
  Gain5/1 -> Add1/4
  Step1/1 -> Product1/2
  Constant4/1 -> Sum/1
  Sum/1 -> Switch/1
  Constant2/1 -> Switch/3
  Constant5/1 -> Sum1/1
  Sum1/1 -> Switch1/1
  Gain4/1 -> Gain6/1, Sum1/2, Sum/2, Switch/2
  Constant3/1 -> Switch1/3
  Gain6/1 -> Switch1/2
  Switch/1 -> Scope1/1, Sum2/1
  Switch1/1 -> Scope3/1, Sum2/2
  Sum2/1 -> Product1/1
  Constant6/1 -> Gain7/1
  Gain7/1 -> Add1/5
  Integrator/1 -> Gain1/1
  Gain/1 -> Out2/1, Scope2/1, Integrator/1
  Product1/1 -> Gain/1
